simulink model "DC_Motor_Buck_Converter"  (R2021a)
settings: Solver=VariableStepAuto  StartTime=0.0  StopTime=2  MaxStep=1e-6  RelTol=1e-3
settings Model: Creator=Shashwat M.A  LastModifiedBy=Shashwat M.A

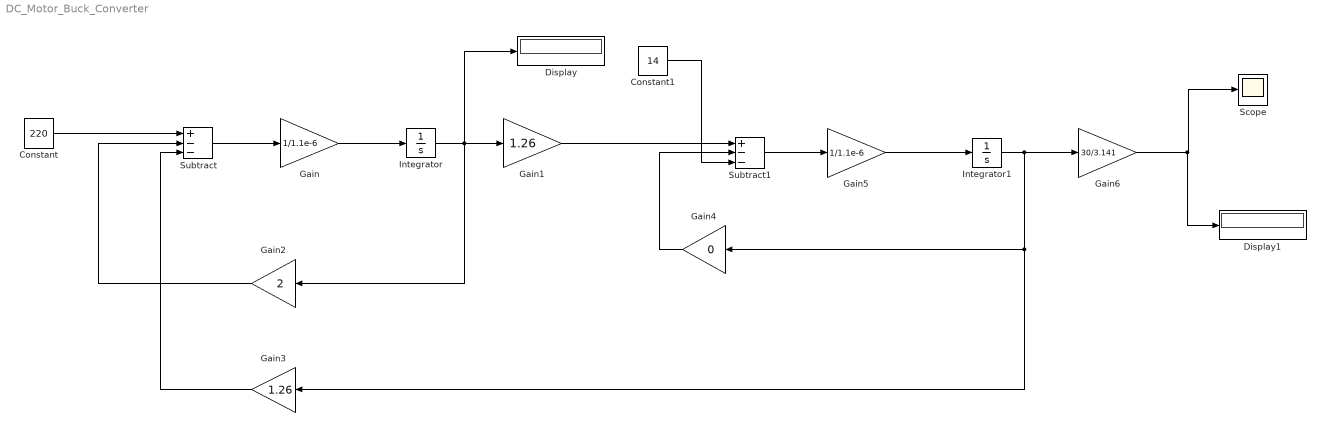
== system DC_Motor_Buck_Converter ==
  Constant : Constant  Value=220
  Constant1 : Constant  Value=14
  Display : Display
  Display1 : Display
  Gain : Gain  Gain=1/1.1e-6
  Gain1 : Gain  Gain=1.26
  Gain2 : Gain  Gain=2
  Gain3 : Gain  Gain=1.26
  Gain4 : Gain  Gain=0
  Gain5 : Gain  Gain=1/1.1e-6
  Gain6 : Gain  Gain=30/3.141
  Integrator : Integrator
  Integrator1 : Integrator
  Scope : Scope
  Subtract : Sum  Inputs=+--
  Subtract1 : Sum  Inputs=+--
  wires:
  Constant/1 -> Subtract/1
  Subtract/1 -> Gain/1
  Gain/1 -> Integrator/1
  Integrator/1 -> Display/1, Gain2/1, Gain1/1
  Gain1/1 -> Subtract1/1
  Gain2/1 -> Subtract/2
  Gain3/1 -> Subtract/3
  Gain4/1 -> Subtract1/2
  Constant1/1 -> Subtract1/3
  Gain5/1 -> Integrator1/1
  Subtract1/1 -> Gain5/1
  Integrator1/1 -> Gain6/1, Gain3/1, Gain4/1
  Gain6/1 -> Display1/1, Scope/1
